simulink library "csc_squ_sequential_update_lib"  (R2014b)
settings: Solver=ode45  SolverMode=SingleTasking  StartTime=0.0  StopTime=10.0  RelTol=1e-3
undefined symbols (not defined in the file or in its folder): kfl_n_meas, kfl_n_state
libraries: simulink x2, util_info_lib x1, csu_mup_measurement_update_lib x1
settings Model: ExtModeAutoUpdateStatusClock=off  Creator=escrane  LastModifiedBy=mstewart

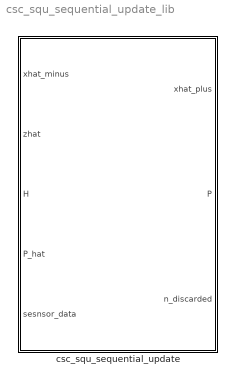
== system csc_squ_sequential_update_lib ==
  csc_squ_sequential_update : Subsystem  TreatAsAtomicUnit=on

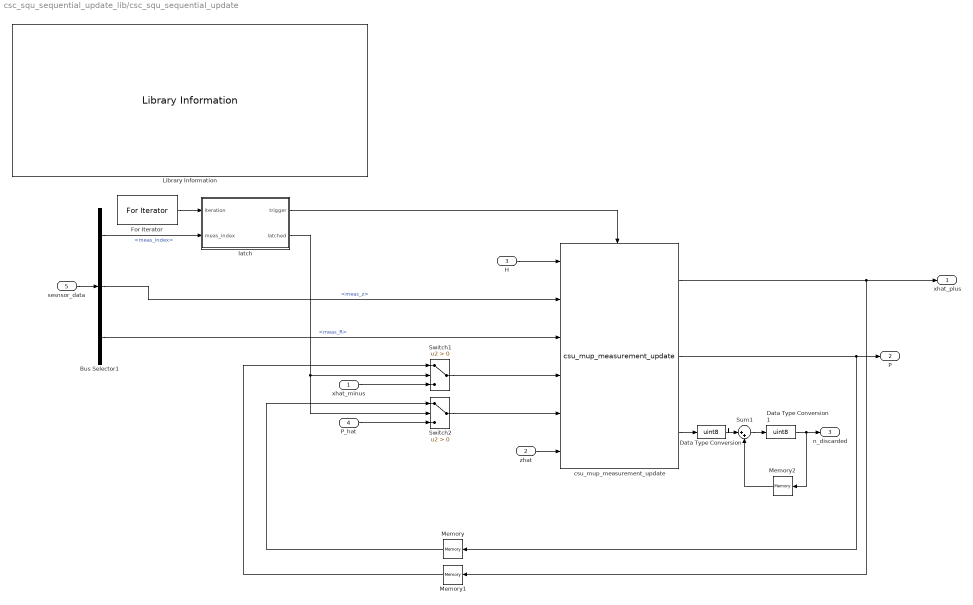
== system csc_squ_sequential_update_lib/csc_squ_sequential_update ==
  xhat_minus : Inport
  zhat : Inport  Port=2
  H : Inport  Port=3
  P_hat : Inport  Port=4
  sesnsor_data : Inport  Port=5
  Bus Selector1 : BusSelector  OutputSignals=meas_index,meas_z,meas_R
  Data Type Conversion : DataTypeConversion  OutDataTypeStr=uint8
  Data Type Conversion1 : DataTypeConversion  OutDataTypeStr=uint8
  For Iterator : ForIterator  ResetStates=reset  IterationLimit=kfl_n_meas
  Library Information : util_info_lib/Library Information  owner='NONE'
  Memory : Memory  X0=zeros(kfl_n_state, kfl_n_state)  InheritSampleTime=on
  Memory1 : Memory  X0=zeros(kfl_n_state,1)  InheritSampleTime=on
  Memory2 : Memory  InheritSampleTime=on
  Sum1 : Sum  Inputs=|++
  Switch1 : Switch  Criteria=u2 > Threshold
  Switch2 : Switch  Criteria=u2 > Threshold
  csu_mup_measurement_update : csu_mup_measurement_update_lib/csu_mup_measurement_update
  latch : Subsystem
  xhat_plus : Outport
  P : Outport  Port=2
  n_discarded : Outport  Port=3
  wires:
  Data Type Conversion1/1 -> n_discarded/1, Memory2/1
  Data Type Conversion/1 -> Sum1/1
  Sum1/1 -> Data Type Conversion1/1
  Memory2/1 -> Sum1/2
  csu_mup_measurement_update/3 -> Data Type Conversion/1
  zhat/1 -> csu_mup_measurement_update/6
  Bus Selector1/3 -> csu_mup_measurement_update/3  "<meas_R>"
  H/1 -> csu_mup_measurement_update/1
  latch/1(trigger) -> csu_mup_measurement_update/Enable
  Bus Selector1/2 -> csu_mup_measurement_update/2  "<meas_z>"
  sesnsor_data/1 -> Bus Selector1/1
  Bus Selector1/1 -> latch/2(meas_index)  "<meas_index>"
  csu_mup_measurement_update/2 -> P/1, Memory/1
  csu_mup_measurement_update/1 -> xhat_plus/1, Memory1/1
  Switch2/1 -> csu_mup_measurement_update/5
  Switch1/1 -> csu_mup_measurement_update/4
  Memory/1 -> Switch2/1
  Memory1/1 -> Switch1/1
  P_hat/1 -> Switch2/3
  xhat_minus/1 -> Switch1/3
  For Iterator/1 -> latch/1(iteration)
  latch/2(latched) -> Switch1/2, Switch2/2

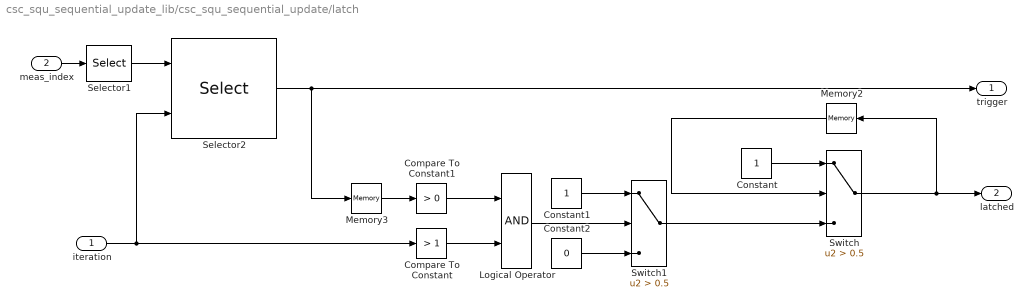
== system csc_squ_sequential_update_lib/csc_squ_sequential_update/latch ==
  iteration : Inport
  meas_index : Inport  Port=2
  Compare To Constant : simulink/Logic and Bit Operations/Compare To Constant  relop=>  const=1  OutDataTypeStr=uint8  ZeroCross=off
  Compare To Constant1 : simulink/Logic and Bit Operations/Compare To Constant  relop=>  const=0  OutDataTypeStr=uint8  ZeroCross=off
  Constant : Constant
  Constant1 : Constant
  Constant2 : Constant  Value=0
  Logical Operator : Logic  AllPortsSameDT=off  OutDataTypeStr=boolean
  Memory2 : Memory  InheritSampleTime=on
  Memory3 : Memory  InheritSampleTime=on
  Selector1 : Selector  InputPortWidth=kfl_n_meas  Indices=[1:kfl_n_meas]
  Selector2 : Selector  InputPortWidth=kfl_n_meas  IndexOptions=Index vector (port)  Indices=[1 3]
  Switch : Switch  Criteria=u2 > Threshold  Threshold=0.5
  Switch1 : Switch  Criteria=u2 > Threshold  Threshold=0.5
  trigger : Outport
  latched : Outport  Port=2
  wires:
  Selector1/1 -> Selector2/1
  Selector2/1 -> Memory3/1, trigger/1
  meas_index/1 -> Selector1/1
  Memory3/1 -> Compare To Constant1/1
  Switch/1 -> Memory2/1, latched/1
  Constant/1 -> Switch/1
  Switch1/1 -> Switch/3
  Memory2/1 -> Switch/2
  iteration/1 -> Selector2/2, Compare To Constant/1
  Compare To Constant/1 -> Logical Operator/2
  Compare To Constant1/1 -> Logical Operator/1
  Logical Operator/1 -> Switch1/2
  Constant1/1 -> Switch1/1
  Constant2/1 -> Switch1/3
